simulink model "rev0BB"  (R2017b)
settings: Solver=FixedStepDiscrete  StartTime=0  StopTime=(((preLen+100+dataLenSymbols)*1+pad_first*3)*basePer)  RelTol=1e-3
values from neighbouring files (symbols this model uses):
  ack_stf_len_symbols = length(x_ACK_STF)    [rev0BB_setup.m]
  agc_delay_lag = 32    [rev0BB_setup.m]
  agc_detector_coef = ones(1,agc_detector_taps)./agc_detector_taps    [rev0BB_setup.m]
  agc_on = true    [rev0BB_startup.m]
  agc_sat_low = -agcSaturation    (= -12)    [rev0BB_setup.m]
  agc_sat_up = agcSaturation    (= 12)    [rev0BB_setup.m]
  agcDesired = 0    [rev0BB_setup.m]
  agcExpDomain = agcSaturation    (= 12)    [rev0BB_setup.m]
  agcExpResolution = 2^-5    (= 0.03125)    [rev0BB_setup.m]
  agcPwrAvgNum = 128    [rev0BB_setup.m]
  agcSaturation = 12    [rev0BB_setup.m]
  agcSettleThresh = 0.65    [rev0BB_setup.m]
  agcStep = 2^-8    (= 0.00390625)    [rev0BB_setup.m]
  atanDomain = 5    [rev0BB_setup.m]
  atanDomainTiming = 256    [rev0BB_setup.m]
  atanResolution = 2^-9    (= 0.001953125)    [rev0BB_setup.m]
  atanResolutionTiming = 2^-5    (= 0.03125)    [rev0BB_setup.m]
  averaging_num = ones(1, averaging_samples)    [rev0BB_setup.m]
  averaging_samples = 128    [rev0BB_setup.m]
  awgnSeed = abs(dBSnrRange(dBSnrInd)*1000+trial+10000000)    [plotBer.m]    (also in rev0BB_startup.m = 67)
  basePer = 1/baseFreq    (= 5e-08)    [rev0BB_setup.m]
  bitsPerSymbolHeader = log2(radixHeader)    [rev0BB_setup.m]
  bitsPerSymbolMax = log2(radixMax)    [rev0BB_setup.m]
  cal_sig_i_mult = 1.0    (= 1)    [rev0BB_startup.m]
  cal_sig_i_offset = 0.0    (= 0)    [rev0BB_startup.m]
  cal_sig_q_mult = 1.0    (= 1)    [rev0BB_startup.m]
  cal_sig_q_offset = 0.0    (= 0)    [rev0BB_startup.m]
  cefEarlyWarning = 256    [rev0BB_setup.m]
  cefLen = length(x_CEF)    [rev0BB_setup.m]
  channelFIR = zeros(1, round(maxSampleDelay)+1)    [rev0BB_startup.m]
  coarseCFOAdaptDelay = 1    [rev0BB_setup.m]
  cr_i = 0.020    (= 0.02)    [rev0BB_setup.m]
  cr_i_preamp = 2^-9    (= 0.001953125)    [rev0BB_setup.m]
  cr_int1_sat_low = -cr_integrator1_saturation    (= -0.6)    [rev0BB_setup.m]
  cr_int1_sat_up = cr_integrator1_saturation    (= 0.6)    [rev0BB_setup.m]
  cr_integrator1_decay = 1    [rev0BB_setup.m]
  cr_integrator1_saturation = 0.6    [rev0BB_setup.m]
  cr_mult_pipeline = 0    [rev0BB_setup.m]
  cr_p = 0.015    [rev0BB_setup.m]
  cr_sat2_low = -cr_saturation2    (= -0.6)    [rev0BB_setup.m]
  cr_sat2_up = cr_saturation2    (= 0.6)    [rev0BB_setup.m]
  cr_smooth_num = (1/cr_smooth_samples).*ones(1, cr_smooth_samples)    [rev0BB_setup.m]
  D_128 = [ 1,  8,  2,  4, 16, 32, 64]    [golay.m]    (also in rev0BB_setup.m)
  D_32 = [ 1,  4,  8,  2, 16]    [golay.m]    (also in rev0BB_setup.m)
  dataLenSymbols = header_len_bytes*8/bitsPerSymbolHeader + frame_len_bytes*8/bitsPerSymbol    [rev0BB_setup.m]
  default_channel = 3    [rev0BB_setup.m]
  dmm_coefs = ones(1,dmm_samples)./dmm_samples    [rev0BB_setup.m]
  dst_field_len = 8    [rev0BB_setup.m]
  expDomain = 3.3    [rev0BB_setup.m]
  expResolution = 2^-5    (= 0.03125)    [rev0BB_setup.m]
  expTol = .1    (= 0.1)    [rev0BB_setup.m]
  flush_delay = regular_pipeline*2+mult_pipeline+4    (= 4)    [rev0BB_setup.m]
  frac_lut_domain = 256    [rev0BB_setup.m]
  frac_lut_domain_cr = 64    [rev0BB_setup.m]
  frac_lut_range_max = 512    [rev0BB_setup.m]
  frac_lut_range_max_coarse_cfo = 127    [rev0BB_setup.m]
  frac_lut_range_max_cr = 127    [rev0BB_setup.m]
  frac_lut_range_min = -frac_lut_range_max    (= -512)    [rev0BB_setup.m]
  frac_lut_range_min_coarse_cfo = -frac_lut_range_max_coarse_cfo    (= -127)    [rev0BB_setup.m]
  frac_lut_range_min_cr = -frac_lut_range_max_cr    (= -127)    [rev0BB_setup.m]
  frac_lut_table_breaks = -frac_lut_domain:frac_lut_res:(frac_lut_domain-1)    [rev0BB_setup.m]
  frac_lut_table_breaks_coarse_cfo = -frac_lut_domain_coarse_cfo:frac_lut_res_coarse_cfo:(frac_lut_domain_coarse_cfo-1)    [rev0BB_setup.m]
  frac_lut_table_breaks_cr = -frac_lut_domain_cr:frac_lut_res_cr:(frac_lut_domain_cr-1)    [rev0BB_setup.m]
  frac_lut_table_data = 1./frac_lut_table_breaks    [rev0BB_setup.m]
  frac_lut_table_data_coarse_cfo = 1./frac_lut_table_breaks_coarse_cfo    [rev0BB_setup.m]
  frac_lut_table_data_cr = 1./frac_lut_table_breaks_cr    [rev0BB_setup.m]
  freeze_en_agc = true    [rev0BB_startup.m]
  freeze_en_cr_int1 = false    [rev0BB_startup.m]
  freeze_en_cr_int2 = false    [rev0BB_startup.m]
  freeze_en_cr_phase = false    [rev0BB_startup.m]
  freeze_en_tr_int1 = false    [rev0BB_startup.m]
  freeze_en_tr_int2 = false    [rev0BB_startup.m]
  freeze_en_tr_phase = false    [rev0BB_startup.m]
  freeze_on_cef_done = true    [rev0BB_startup.m]
  freeze_on_stf_done = false    [rev0BB_startup.m]
  freeze_on_valid = true    [rev0BB_startup.m]
  golay_type = 32    [rev0BB_setup.m]
  guardInt = int16(4)    [rev0BB_setup.m]
  guardTol = int16(5)    [rev0BB_setup.m]
  header_len_bytes = 8    [rev0BB_setup.m]
  lineWidth = 60    [rev0BB_setup.m]
  lmsEqDepth = 38    [rev0BB_setup.m]
  lmsStep_init = 0.006    [rev0BB_setup.m]
  lmsStep_meta = (lmsStep_final - lmsStep_init)/cefLen    [rev0BB_setup.m]
  lnDomain = 16    [rev0BB_setup.m]
  lnResolution = 2^-5    (= 0.03125)    [rev0BB_setup.m]
  local_node_id = 2    [rev0BB_startup.m]
  maxMsgSize = length(xSpectrum_PRE)+dataLenSymbols+300    [rev0BB_setup.m]
  minSTFPeaks = 3    [rev0BB_setup.m]
  mod_scheme_len_bytes = 1    [rev0BB_setup.m]
  modBPS = [1, 2, 4]    [rev0BB_setup.m]
  modKeys = [0, 1, 2]    [rev0BB_setup.m]
  mult_pipeline = 0    [rev0BB_setup.m]
  overSampleFreq = 80e6    (= 80000000)    [rev0BB_setup.m]
  overSamplePer = 1/overSampleFreq    (= 1.25e-08)    [rev0BB_setup.m]
  pad_first = 1000    [createTestVectors.m]
  post_cr_i_offset = 0    [rev0BB_startup.m]
  post_cr_q_offset = 0    [rev0BB_startup.m]
  preambleSequentialDetect = 2    [rev0BB_setup.m]
  preLen = length(x_PRE)    [rev0BB_setup.m]
  qam16_demod_scale_factor = qam16_hdl_distance/qam16_power_normalized_distance    [rev0BB_setup.m]
  rcRxFilt = [0.000303163120401141 -0.00118915940834234 -0.00187387637177 -0.00124167532697737 0.00029186889076529 0.00164526160586517 0.00182432050803312 0.000652133621739543 -0.00105668254004908 -0.00204011570659167 -0.00150058088768918 0.00026138356356816 0.0019831869994874 0.00231075800085521 0.000821993419120097 -0.00154687337975486 -0.00305430783933469 -0.00238186490079127 0.000301216962040692 0.00325307 ...(+2001 chars)    [rev0BB_setup.m]
  rcTxFilt = [0.000303163120401141 -0.00118915940834234 -0.00187387637177 -0.00124167532697737 0.00029186889076529 0.00164526160586517 0.00182432050803312 0.000652133621739543 -0.00105668254004908 -0.00204011570659167 -0.00150058088768918 0.00026138356356816 0.0019831869994874 0.00231075800085521 0.000821993419120097 -0.00154687337975486 -0.00305430783933469 -0.00238186490079127 0.000301216962040692 0.00325307 ...(+2001 chars)    [rev0BB_setup.m]
  regular_pipeline = 0    [rev0BB_setup.m]
  rx_gain = 1    [rev0BB_setup.m]
  rx_gain_i = 1    [rev0BB_setup.m]
  rx_gain_q = 1    [rev0BB_setup.m]
  rx_impare_i_offset = 0    [rev0BB_startup.m]
  rx_impare_i_scale = 1    [rev0BB_startup.m]
  rx_impare_q_offset = 0    [rev0BB_startup.m]
  rx_impare_q_scale = 1    [rev0BB_startup.m]
  rx_offset_correction_i = 0    [rev0BB_startup.m]
  rx_offset_correction_q = 0    [rev0BB_startup.m]
  sin_source_amp = 1    [rev0BB_setup.m]
  sin_source_freq = 250e6/16    (= 15625000)    [rev0BB_setup.m]
  slowPer = overSamplePer*slowSample    (= 2.5e-08)    [rev0BB_setup.m]
  std_pkt_type = 0    [rev0BB_setup.m]
  stfLen = length(x_STF)    [rev0BB_setup.m]
  testMsg = cat(1, xCTRL_PRE_adj, header, payload)    [plotBer.m]
  timing_i = 0.25    [rev0BB_setup.m]
  ... (+25 more)
undefined symbols (not defined in the file or in its folder): cr_integrator2_saturation, doppler, i, magnitude, useFadingChannel
libraries: helperLib x128, simulink x90, golayLib x34, dspsigops x32, commfilt2 x27, commdigbbndpm3 x8, hdlsllib x6, dsparch4 x4, commdigbbndam3 x4, commchan3 x2, commrflib2 x2, commcrc2 x2
(part 5 of 10)

== system rev0BB/receiver/fast_rx_baseband/Timing Recovery/SampleAccum ==
  note: Based on Digital Communication Recievers by Meyr pg 530 but modified
      |
      | The error here is in "samples". The correction input is in fact -error and
      | dictates how the clock should be changed.
      |
      | The clk_per is not simply the integer portion of the delay, which is
      | somewhat counterintuitive. This is because the clk_per line is controling
      | the delay for the rx clk (in terms of samples). Here is some intuition:
      | Say that the desired phase is exactly on a sample (fractional delay = 0).
      | One can get the same phase by setting the fractional phase to 1 but the
      | clock must add 1 sample to catch up with the additional delay added.
      |
      | The same logic holds true in the reverse case. Delay can be changed
      | from 1 to 0 but the clock must skip a sample to catch up.
      |
      | Diagrams showing the clock logic as well as the logic when a phase correction
      | is non-zeros are presented to the left of this text.
  note: Division Represented as Shift
  correction : Inport
  Enable : EnablePort
  Add1 : Sum  OutDataTypeStr=Inherit: Same as first input
  Add2 : Sum  OutDataTypeStr=Inherit: Same as first input
  Add4 : Sum  OutDataTypeStr=Inherit: Same as first input
  Constant3 : Constant  Value=4  OutDataTypeStr=Inherit: Inherit via back propagation  SampleTime=-1
  Constant4 : Constant  Value=4  OutDataTypeStr=Inherit: Inherit via back propagation  SampleTime=-1
  Data Type Conversion1 : DataTypeConversion  OutDataTypeStr=int8
  Data Type Conversion2 : DataTypeConversion
  Data Type Conversion3 : DataTypeConversion
  Delay2 : Delay  DelayLength=1  InitialCondition=0
  Gain : Gain  Gain=-1  OutDataTypeStr=Inherit: Same as input
  Sub2 : Sum  Inputs=+-  OutDataTypeStr=Inherit: Same as first input
  Sub3 : Sum  Inputs=+-  OutDataTypeStr=Inherit: Same as first input
  fracDelay : Outport  InitialOutput=[0]
  clk_per : Outport  Port=2  InitialOutput=[0]
  fullDelay : Outport  Port=3  InitialOutput=[0]
  wires:
  Sub3/1 -> Gain/1
  Constant3/1 -> Add1/2
  Data Type Conversion1/1 -> Sub3/1, Data Type Conversion2/1
  Delay2/1 -> Add2/2
  Add2/1 -> fullDelay/1, Data Type Conversion3/1, Data Type Conversion1/1
  Add4/1 -> clk_per/1
  Constant4/1 -> Add4/2, Sub3/2
  correction/1 -> Add1/1
  Gain/1 -> Add4/1
  Sub2/1 -> fracDelay/1, Delay2/1
  Add1/1 -> Add2/1
  Data Type Conversion2/1 -> Sub2/2
  Data Type Conversion3/1 -> Sub2/1

== system rev0BB/receiver/fast_rx_baseband/Timing Recovery/frac_delay_farrow_N-2_M-3 ==
  note: 1
  note: 3
  note: 1
  note: 3
  note: 1
  note: 3
  note: Based on Digital Communication Receivers by Meyr pg 515, 521-522
  note: Delays contained in FIR
  samples : Inport
  delay : Inport  Port=2
  Add : Sum  OutDataTypeStr=Inherit: Same as first input
  Add1 : Sum  OutDataTypeStr=Inherit: Same as first input
  Add2 : Sum  OutDataTypeStr=Inherit: Same as first input
  Discrete FIR Filter : DiscreteFir  FilterStructure=Direct form transposed  Coefficients=[-0.22485, 0.64567, -0.64567, 0.22485]  OutDataTypeStr=Inherit: Same as input
  Discrete FIR Filter1 : DiscreteFir  FilterStructure=Direct form transposed  Coefficients=[0.70609, -1.31155, 0.62547, 0.03154]  OutDataTypeStr=Inherit: Same as input
  Discrete FIR Filter2 : DiscreteFir  FilterStructure=Direct form transposed  Coefficients=[-0.48124, -0.33413, 1.02020, -0.25639]  OutDataTypeStr=Inherit: Same as input
  Discrete FIR Filter3 : DiscreteFir  FilterStructure=Direct form transposed  Coefficients=[0, 1, 0, 0]  OutDataTypeStr=Inherit: Same as input
  Product1 : Product  OutDataTypeStr=Inherit: Same as first input
  Product2 : Product  OutDataTypeStr=Inherit: Same as first input
  Product5 : Product  OutDataTypeStr=Inherit: Same as first input
  mult_delay{,1..5} (6 alike) : Delay  DelayLength=mult_pipeline
  mult_delay_match : Delay  DelayLength=mult_pipeline
  mult_delay_match1 : Delay  DelayLength=mult_pipeline
  mult_delay_match2 : Delay  DelayLength=mult_pipeline
  mult_delay_match3 : Delay  DelayLength=mult_pipeline*2
  mult_delay_match4 : Delay  DelayLength=mult_pipeline*3
  pipeline_delay{,1..10} (11 alike) : Delay  DelayLength=regular_pipeline
  pipeline_delay_match : Delay  DelayLength=regular_pipeline
  pipeline_delay_match1 : Delay  DelayLength=regular_pipeline
  pipeline_delay_match2 : Delay  DelayLength=regular_pipeline
  pipeline_delay_match3 : Delay  DelayLength=regular_pipeline*2
  out : Outport
  wires:
  Discrete FIR Filter3/1 -> pipeline_delay9/1
  Discrete FIR Filter/1 -> pipeline_delay6/1
  delay/1 -> mult_delay3/1, mult_delay_match/1
  samples/1 -> pipeline_delay10/1
  Discrete FIR Filter1/1 -> pipeline_delay7/1
  Product5/1 -> pipeline_delay3/1
  Add/1 -> mult_delay1/1
  Discrete FIR Filter2/1 -> pipeline_delay8/1
  Add1/1 -> mult_delay2/1
  Add2/1 -> out/1
  Product1/1 -> pipeline_delay4/1
  Product2/1 -> pipeline_delay5/1
  mult_delay_match/1 -> pipeline_delay_match/1
  mult_delay_match1/1 -> pipeline_delay_match1/1
  mult_delay_match2/1 -> pipeline_delay/1
  mult_delay_match3/1 -> pipeline_delay_match2/1
  mult_delay_match4/1 -> pipeline_delay_match3/1
  mult_delay3/1 -> Product5/2
  mult_delay/1 -> Product5/1
  mult_delay1/1 -> Product1/1
  mult_delay4/1 -> Product1/2
  mult_delay2/1 -> Product2/1
  mult_delay5/1 -> Product2/2
  pipeline_delay/1 -> Add/1
  pipeline_delay3/1 -> Add/2
  pipeline_delay4/1 -> Add1/2
  pipeline_delay5/1 -> Add2/2
  pipeline_delay_match/1 -> mult_delay_match1/1, mult_delay4/1
  pipeline_delay_match1/1 -> mult_delay5/1
  pipeline_delay6/1 -> mult_delay/1
  pipeline_delay7/1 -> mult_delay_match2/1
  pipeline_delay8/1 -> mult_delay_match3/1
  pipeline_delay9/1 -> mult_delay_match4/1
  pipeline_delay10/1 -> Discrete FIR Filter/1, Discrete FIR Filter1/1, Discrete FIR Filter2/1, Discrete FIR Filter3/1
  pipeline_delay1/1 -> Add1/1
  pipeline_delay_match2/1 -> pipeline_delay1/1
  pipeline_delay2/1 -> Add2/1
  pipeline_delay_match3/1 -> pipeline_delay2/1

== system rev0BB/receiver/fast_rx_baseband/Timing Recovery/loopFilter ==
  In : Inport
  timing_p : Inport  Port=2
  timing_i : Inport  Port=3
  timing_integrator1_decay : Inport  Port=4
  tr_int1_sat_up : Inport  Port=5
  tr_int1_sat_low : Inport  Port=6
  int1_freeze : Inport  Port=7  OutDataTypeStr=boolean
  timing_pre_scale : Inport  Port=8
  tr_sat2_up : Inport  Port=9
  tr_sat2_low : Inport  Port=10
  Enable : EnablePort
  Add : Sum  OutDataTypeStr=Inherit: Same as first input
  Add1 : Sum  OutDataTypeStr=Inherit: Same as first input
  Constant : Constant  Value=0  OutDataTypeStr=Inherit: Inherit via back propagation  SampleTime=-1
  Data Type Duplicate{,1..2,4} (4 alike) : DataTypeDuplicate
  Data Type Conversion4 : DataTypeConversion  OutDataTypeStr=single
  Delay1 : Delay  DelayLength=1  InitialCondition=0
  Delay12 : Delay  DelayLength=1
  Discrete FIR Filter : DiscreteFir  FilterStructure=Direct form transposed  Coefficients=timing_smooth_num  OutDataTypeStr=Inherit: Same as input
  Switch1 : Switch  Criteria=u2 > Threshold
  Switch2 : Switch  Criteria=u2 > Threshold
  pipeline_delay1 : Delay  DelayLength=regular_pipeline
  pipeline_delay5 : Delay  DelayLength=regular_pipeline
  pipeline_delay9 : Delay  DelayLength=regular_pipeline
  pipelined_mult{,1..3} (4 alike) : helperLib/pipelined_mult  d=wide_mult_pipeline
  sat : Subsystem
  sat1 : Subsystem
  Out : Outport  InitialOutput=0
  wires:
  In/1 -> pipeline_delay5/1
  Discrete FIR Filter/1 -> pipeline_delay1/1
  Add/1 -> sat/1(In1)
  sat1/1(Out1) -> Data Type Conversion4/1
  pipelined_mult3/1 -> Switch1/3
  Data Type Conversion4/1 -> Out/1
  pipelined_mult2/1 -> Delay12/1
  Switch2/1 -> Add1/1
  timing_p/1 -> Data Type Duplicate4/1, Data Type Duplicate4/2, pipelined_mult1/2
  timing_integrator1_decay/1 -> Data Type Duplicate/2, pipelined_mult2/1
  timing_i/1 -> pipelined_mult3/2, Data Type Duplicate1/2
  Add1/1 -> pipeline_delay9/1
  tr_int1_sat_up/1 -> sat/2(limit_up)
  tr_int1_sat_low/1 -> sat/3(limit_low)
  Delay1/1 -> Switch1/1
  int1_freeze/1 -> Switch2/2, Switch1/2
  Switch1/1 -> Delay1/1, Add1/2
  pipelined_mult1/1 -> Switch2/3
  Constant/1 -> Switch2/1
  sat/1(Out1) -> Data Type Duplicate1/1, pipelined_mult3/1, Data Type Duplicate/1, pipelined_mult2/2
  pipeline_delay1/1 -> pipelined_mult/1, Data Type Duplicate2/1, pipelined_mult1/1
  timing_pre_scale/1 -> Data Type Duplicate2/2, pipelined_mult/2
  pipeline_delay5/1 -> Discrete FIR Filter/1
  pipelined_mult/1 -> Add/1
  tr_sat2_up/1 -> sat1/2(limit_up)
  tr_sat2_low/1 -> sat1/3(limit_low)
  pipeline_delay9/1 -> sat1/1(In1)
  Delay12/1 -> Add/2

== system rev0BB/receiver/fast_rx_baseband/Timing Recovery/nda_4x_time_err_enable ==
  note: Design from Digital Communication Recievers by Meyr. pg 291, 529
  samples : Inport
  enable : Inport  Port=2
  phase_est : Subsystem
  "tapped_delay4 " : Subsystem  AncestorBlock=helperLib/tapped_delay4
  err : Outport
  wires:
  "tapped_delay4 "/3(delay_1) -> phase_est/3(In3)
  "tapped_delay4 "/4(delay_0) -> phase_est/4(In4)
  "tapped_delay4 "/1(delay_3) -> phase_est/1(In1)
  "tapped_delay4 "/2(delay_2) -> phase_est/2(In2)
  phase_est/1(Out1) -> err/1
  enable/1 -> phase_est/Enable
  samples/1 -> "tapped_delay4 "/1(symbol)

== system rev0BB/receiver/fast_rx_baseband/Timing Recovery/sat ==
  In1 : Inport
  Saturation : Saturate  UpperLimit=.5  LowerLimit=-.5
  Out1 : Outport
  wires:
  Saturation/1 -> Out1/1
  In1/1 -> Saturation/1

== system rev0BB/receiver/slim_fast_rx/AGC/exp ==
  note: Bound Protection
  In : Inport
  Compare To Constant1 : simulink/Logic and Bit Operations/Compare To Constant  relop=>=  const=agcExpDomain  OutDataTypeStr=boolean
  Compare To Constant4 : simulink/Logic and Bit Operations/Compare To Constant  relop=<=  const=-agcExpDomain  OutDataTypeStr=boolean
  Constant11 : Constant  Value=0  OutDataTypeStr=Inherit: Inherit via back propagation  SampleTime=-1
  Constant3 : Constant  Value=exp(agcExpDomain)  OutDataTypeStr=Inherit: Inherit via back propagation  SampleTime=-1
  Constant4 : Constant  Value=exp(-agcExpDomain)  OutDataTypeStr=Inherit: Inherit via back propagation  SampleTime=-1
  Data Type Duplicate : DataTypeDuplicate
  Data Type Duplicate1 : DataTypeDuplicate
  Data Type Duplicate2 : DataTypeDuplicate
  Data Type Conversion : DataTypeConversion  OutDataTypeStr=fixdt(1,ceil(log2(agcExpDomain))-floor(log2(agcExpResolution))+2,-floor(log2(agcExpResolution)))
  Logical Operator : Logic  Operator=OR  AllPortsSameDT=off  OutDataTypeStr=boolean
  Switch2 : Switch  Criteria=u2 ~= 0  OutDataTypeStr=Inherit: Inherit via back propagation
  Switch3 : Switch  Criteria=u2 ~= 0  OutDataTypeStr=Inherit: Inherit via back propagation
  Switch8 : Switch  Criteria=u2 ~= 0  OutDataTypeStr=Inherit: Inherit via back propagation
  exp Lookup Table : Lookup_n-D  NumberOfTableDimensions=1  BreakpointsForDimension1=[-agcExpDomain:agcExpResolution:agcExpDomain]  IndexSearchMethod=Evenly spaced points  Table=exp([-agcExpDomain:agcExpResolution:agcExpDomain])  InterpMethod=Flat  DiagnosticForOutOfRangeInput=Error  RemoveProtectionInput=on  InternalRulePriority=Speed  OutDataTypeStr=Inherit: Inherit via back propagation  RndMeth=Simplest  InputSameDT=on
  pipeline_delay1 : Delay  DelayLength=regular_pipeline
  pipeline_delay2 : Delay  DelayLength=regular_pipeline  InitialCondition=1
  pipeline_delay_match : Delay  DelayLength=regular_pipeline*2
  pipeline_delay_match1 : Delay  DelayLength=regular_pipeline*2
  Out : Outport
  wires:
  pipeline_delay2/1 -> Data Type Duplicate2/1, Switch2/3
  pipeline_delay1/1 -> exp Lookup Table/1
  pipeline_delay_match1/1 -> Switch3/2
  pipeline_delay_match/1 -> Switch2/2
  exp Lookup Table/1 -> Data Type Duplicate/2, pipeline_delay2/1
  Constant11/1 -> Switch8/1
  Logical Operator/1 -> Switch8/2
  Switch3/1 -> Data Type Duplicate1/2, Data Type Duplicate2/2, Out/1
  Constant4/1 -> Switch3/1
  Switch2/1 -> Data Type Duplicate1/1, Switch3/3
  Constant3/1 -> Switch2/1
  Compare To Constant4/1 -> pipeline_delay_match1/1, Logical Operator/2
  Compare To Constant1/1 -> pipeline_delay_match/1, Logical Operator/1
  In/1 -> Data Type Duplicate/1, Compare To Constant4/1, Compare To Constant1/1, Switch8/3
  Switch8/1 -> Data Type Conversion/1
  Data Type Conversion/1 -> pipeline_delay1/1

== system rev0BB/receiver/slim_fast_rx/AGC/exp1 ==
  note: Bound Protection
  In : Inport
  Compare To Constant1 : simulink/Logic and Bit Operations/Compare To Constant  relop=>=  const=agcExpDomain*2  OutDataTypeStr=boolean
  Compare To Constant4 : simulink/Logic and Bit Operations/Compare To Constant  relop=<=  const=-agcExpDomain*2  OutDataTypeStr=boolean
  Constant11 : Constant  Value=0  OutDataTypeStr=Inherit: Inherit via back propagation  SampleTime=-1
  Constant3 : Constant  Value=exp(agcExpDomain*2)  OutDataTypeStr=Inherit: Inherit via back propagation  SampleTime=-1
  Constant4 : Constant  Value=exp(-agcExpDomain)  OutDataTypeStr=Inherit: Inherit via back propagation  SampleTime=-1
  Data Type Duplicate : DataTypeDuplicate
  Data Type Duplicate1 : DataTypeDuplicate
  Data Type Duplicate2 : DataTypeDuplicate
  Data Type Conversion : DataTypeConversion  OutDataTypeStr=fixdt(1,ceil(log2(agcExpDomain*2))-floor(log2(agcExpResolution))+2,-floor(log2(agcExpResolution)))
  Logical Operator : Logic  Operator=OR  AllPortsSameDT=off  OutDataTypeStr=boolean
  Switch2 : Switch  Criteria=u2 ~= 0  OutDataTypeStr=Inherit: Inherit via back propagation
  Switch3 : Switch  Criteria=u2 ~= 0  OutDataTypeStr=Inherit: Inherit via back propagation
  Switch8 : Switch  Criteria=u2 ~= 0  OutDataTypeStr=Inherit: Inherit via back propagation
  exp Lookup Table : Lookup_n-D  NumberOfTableDimensions=1  BreakpointsForDimension1=[(-agcExpDomain*2):agcExpResolution:agcExpDomain*2]  IndexSearchMethod=Evenly spaced points  Table=exp([(-agcExpDomain*2):agcExpResolution:(agcExpDomain*2)])  InterpMethod=Flat  DiagnosticForOutOfRangeInput=Error  RemoveProtectionInput=on  InternalRulePriority=Speed  OutDataTypeStr=Inherit: Inherit via back propagation  RndMeth=Simplest  InputSameDT=on
  mult_delay : Delay  DelayLength=wide_mult_pipeline
  mult_delay_match : Delay  DelayLength=wide_mult_pipeline
  mult_delay_match1 : Delay  DelayLength=wide_mult_pipeline
  pipeline_delay1 : Delay  DelayLength=regular_pipeline
  pipeline_delay2 : Delay  DelayLength=regular_pipeline  InitialCondition=1
  pipeline_delay_match : Delay  DelayLength=regular_pipeline*2
  pipeline_delay_match1 : Delay  DelayLength=regular_pipeline*2
  Out : Outport
  wires:
  pipeline_delay2/1 -> Switch2/3, Data Type Duplicate2/2
  mult_delay/1 -> exp Lookup Table/1
  pipeline_delay1/1 -> mult_delay/1
  mult_delay_match1/1 -> Switch3/2
  mult_delay_match/1 -> Switch2/2
  pipeline_delay_match1/1 -> mult_delay_match1/1
  pipeline_delay_match/1 -> mult_delay_match/1
  exp Lookup Table/1 -> Data Type Duplicate/2, pipeline_delay2/1
  Switch8/1 -> Data Type Conversion/1
  Constant11/1 -> Switch8/1
  Logical Operator/1 -> Switch8/2
  Switch3/1 -> Data Type Duplicate2/1, Data Type Duplicate1/2, Out/1
  Constant4/1 -> Switch3/1
  Switch2/1 -> Data Type Duplicate1/1, Switch3/3
  Constant3/1 -> Switch2/1
  Compare To Constant4/1 -> pipeline_delay_match1/1, Logical Operator/2
  Compare To Constant1/1 -> pipeline_delay_match/1, Logical Operator/1
  In/1 -> Data Type Duplicate/1, Compare To Constant4/1, Compare To Constant1/1, Switch8/3
  Data Type Conversion/1 -> pipeline_delay1/1

== system rev0BB/receiver/slim_fast_rx/AGC/ln1 ==
  note: Note that output type is scaled back
  note: Bound Protection
  In : Inport
  data_type : Inport  Port=2
  Compare To Constant1 : simulink/Logic and Bit Operations/Compare To Constant  relop=>=  const=lnDomain  OutDataTypeStr=boolean
  Compare To Constant4 : simulink/Logic and Bit Operations/Compare To Constant  relop=<=  const=lnResolution  OutDataTypeStr=boolean
  Constant11 : Constant  Value=lnResolution  OutDataTypeStr=Inherit: Inherit via back propagation  SampleTime=-1
  Constant3 : Constant  Value=log(lnDomain)  OutDataTypeStr=Inherit: Inherit via back propagation  SampleTime=-1
  Constant4 : Constant  Value=log(lnResolution)  OutDataTypeStr=Inherit: Inherit via back propagation  SampleTime=-1
  Data Type Duplicate : DataTypeDuplicate
  Data Type Conversion : DataTypeConversion  OutDataTypeStr=single
  Logical Operator : Logic  Operator=OR  AllPortsSameDT=off  OutDataTypeStr=boolean
  Saturation : Saturate  UpperLimit=lnDomain  LowerLimit=lnResolution
  Switch2 : Switch  Criteria=u2 ~= 0  OutDataTypeStr=Inherit: Inherit via back propagation
  Switch3 : Switch  Criteria=u2 ~= 0  OutDataTypeStr=Inherit: Inherit via back propagation
  Switch8 : Switch  Criteria=u2 ~= 0  OutDataTypeStr=Inherit: Inherit via back propagation
  ln Lookup Table : Lookup_n-D  NumberOfTableDimensions=1  BreakpointsForDimension1=[lnResolution:lnResolution:lnDomain]  IndexSearchMethod=Evenly spaced points  Table=log([lnResolution:lnResolution:lnDomain])  InterpMethod=Flat  DiagnosticForOutOfRangeInput=Error  RemoveProtectionInput=on  InternalRulePriority=Speed  OutDataTypeStr=Inherit: Inherit via back propagation  RndMeth=Simplest  InputSameDT=on
  pipeline_delay1 : Delay  DelayLength=regular_pipeline  InitialCondition=0
  pipeline_delay2 : Delay  DelayLength=regular_pipeline*2
  pipeline_delay3 : Delay  DelayLength=regular_pipeline*1  InitialCondition=1
  pipeline_delay_match : Delay  DelayLength=regular_pipeline*4
  pipeline_delay_match1 : Delay  DelayLength=regular_pipeline*4
  Out : Outport
  wires:
  pipeline_delay2/1 -> Switch2/3
  pipeline_delay1/1 -> Saturation/1
  pipeline_delay_match1/1 -> Switch3/2
  pipeline_delay_match/1 -> Switch2/2
  ln Lookup Table/1 -> Data Type Duplicate/2, pipeline_delay2/1
  Constant11/1 -> Switch8/1
  Logical Operator/1 -> Switch8/2
  Switch3/1 -> Out/1
  Constant4/1 -> Switch3/1
  Switch2/1 -> Switch3/3
  Constant3/1 -> Switch2/1
  Compare To Constant4/1 -> pipeline_delay_match1/1, Logical Operator/2
  Compare To Constant1/1 -> pipeline_delay_match/1, Logical Operator/1
  Saturation/1 -> pipeline_delay3/1
  pipeline_delay3/1 -> ln Lookup Table/1
  In/1 -> Compare To Constant4/1, Compare To Constant1/1, Switch8/3
  data_type/1 -> Data Type Duplicate/1
  Switch8/1 -> Data Type Conversion/1
  Data Type Conversion/1 -> pipeline_delay1/1

== system rev0BB/receiver/slim_fast_rx1/AGC/exp ==
  note: Bound Protection
  In : Inport
  Compare To Constant1 : simulink/Logic and Bit Operations/Compare To Constant  relop=>=  const=agcExpDomain  OutDataTypeStr=boolean
  Compare To Constant4 : simulink/Logic and Bit Operations/Compare To Constant  relop=<=  const=-agcExpDomain  OutDataTypeStr=boolean
  Constant11 : Constant  Value=0  OutDataTypeStr=Inherit: Inherit via back propagation  SampleTime=-1
  Constant3 : Constant  Value=exp(agcExpDomain)  OutDataTypeStr=Inherit: Inherit via back propagation  SampleTime=-1
  Constant4 : Constant  Value=exp(-agcExpDomain)  OutDataTypeStr=Inherit: Inherit via back propagation  SampleTime=-1
  Data Type Duplicate : DataTypeDuplicate
  Data Type Duplicate1 : DataTypeDuplicate
  Data Type Duplicate2 : DataTypeDuplicate
  Data Type Conversion : DataTypeConversion  OutDataTypeStr=fixdt(1,ceil(log2(agcExpDomain))-floor(log2(agcExpResolution))+2,-floor(log2(agcExpResolution)))
  Logical Operator : Logic  Operator=OR  AllPortsSameDT=off  OutDataTypeStr=boolean
  Switch2 : Switch  Criteria=u2 ~= 0  OutDataTypeStr=Inherit: Inherit via back propagation
  Switch3 : Switch  Criteria=u2 ~= 0  OutDataTypeStr=Inherit: Inherit via back propagation
  Switch8 : Switch  Criteria=u2 ~= 0  OutDataTypeStr=Inherit: Inherit via back propagation
  exp Lookup Table : Lookup_n-D  NumberOfTableDimensions=1  BreakpointsForDimension1=[-agcExpDomain:agcExpResolution:agcExpDomain]  IndexSearchMethod=Evenly spaced points  Table=exp([-agcExpDomain:agcExpResolution:agcExpDomain])  InterpMethod=Flat  DiagnosticForOutOfRangeInput=Error  RemoveProtectionInput=on  InternalRulePriority=Speed  OutDataTypeStr=Inherit: Inherit via back propagation  RndMeth=Simplest  InputSameDT=on
  pipeline_delay1 : Delay  DelayLength=regular_pipeline
  pipeline_delay2 : Delay  DelayLength=regular_pipeline  InitialCondition=1
  pipeline_delay_match : Delay  DelayLength=regular_pipeline*2
  pipeline_delay_match1 : Delay  DelayLength=regular_pipeline*2
  Out : Outport
  wires:
  pipeline_delay2/1 -> Data Type Duplicate2/1, Switch2/3
  pipeline_delay1/1 -> exp Lookup Table/1
  pipeline_delay_match1/1 -> Switch3/2
  pipeline_delay_match/1 -> Switch2/2
  exp Lookup Table/1 -> Data Type Duplicate/2, pipeline_delay2/1
  Constant11/1 -> Switch8/1
  Logical Operator/1 -> Switch8/2
  Switch3/1 -> Data Type Duplicate1/2, Data Type Duplicate2/2, Out/1
  Constant4/1 -> Switch3/1
  Switch2/1 -> Data Type Duplicate1/1, Switch3/3
  Constant3/1 -> Switch2/1
  Compare To Constant4/1 -> pipeline_delay_match1/1, Logical Operator/2
  Compare To Constant1/1 -> pipeline_delay_match/1, Logical Operator/1
  In/1 -> Data Type Duplicate/1, Compare To Constant4/1, Compare To Constant1/1, Switch8/3
  Switch8/1 -> Data Type Conversion/1
  Data Type Conversion/1 -> pipeline_delay1/1

== system rev0BB/receiver/slim_fast_rx1/AGC/exp1 ==
  note: Bound Protection
  In : Inport
  Compare To Constant1 : simulink/Logic and Bit Operations/Compare To Constant  relop=>=  const=agcExpDomain*2  OutDataTypeStr=boolean
  Compare To Constant4 : simulink/Logic and Bit Operations/Compare To Constant  relop=<=  const=-agcExpDomain*2  OutDataTypeStr=boolean
  Constant11 : Constant  Value=0  OutDataTypeStr=Inherit: Inherit via back propagation  SampleTime=-1
  Constant3 : Constant  Value=exp(agcExpDomain*2)  OutDataTypeStr=Inherit: Inherit via back propagation  SampleTime=-1
  Constant4 : Constant  Value=exp(-agcExpDomain)  OutDataTypeStr=Inherit: Inherit via back propagation  SampleTime=-1
  Data Type Duplicate : DataTypeDuplicate
  Data Type Duplicate1 : DataTypeDuplicate
  Data Type Duplicate2 : DataTypeDuplicate
  Data Type Conversion : DataTypeConversion  OutDataTypeStr=fixdt(1,ceil(log2(agcExpDomain*2))-floor(log2(agcExpResolution))+2,-floor(log2(agcExpResolution)))
  Logical Operator : Logic  Operator=OR  AllPortsSameDT=off  OutDataTypeStr=boolean
  Switch2 : Switch  Criteria=u2 ~= 0  OutDataTypeStr=Inherit: Inherit via back propagation
  Switch3 : Switch  Criteria=u2 ~= 0  OutDataTypeStr=Inherit: Inherit via back propagation
  Switch8 : Switch  Criteria=u2 ~= 0  OutDataTypeStr=Inherit: Inherit via back propagation
  exp Lookup Table : Lookup_n-D  NumberOfTableDimensions=1  BreakpointsForDimension1=[(-agcExpDomain*2):agcExpResolution:agcExpDomain*2]  IndexSearchMethod=Evenly spaced points  Table=exp([(-agcExpDomain*2):agcExpResolution:(agcExpDomain*2)])  InterpMethod=Flat  DiagnosticForOutOfRangeInput=Error  RemoveProtectionInput=on  InternalRulePriority=Speed  OutDataTypeStr=Inherit: Inherit via back propagation  RndMeth=Simplest  InputSameDT=on
  mult_delay : Delay  DelayLength=wide_mult_pipeline
  mult_delay_match : Delay  DelayLength=wide_mult_pipeline
  mult_delay_match1 : Delay  DelayLength=wide_mult_pipeline
  pipeline_delay1 : Delay  DelayLength=regular_pipeline
  pipeline_delay2 : Delay  DelayLength=regular_pipeline  InitialCondition=1
  pipeline_delay_match : Delay  DelayLength=regular_pipeline*2
  pipeline_delay_match1 : Delay  DelayLength=regular_pipeline*2
  Out : Outport
  wires:
  pipeline_delay2/1 -> Switch2/3, Data Type Duplicate2/2
  mult_delay/1 -> exp Lookup Table/1
  pipeline_delay1/1 -> mult_delay/1
  mult_delay_match1/1 -> Switch3/2
  mult_delay_match/1 -> Switch2/2
  pipeline_delay_match1/1 -> mult_delay_match1/1
  pipeline_delay_match/1 -> mult_delay_match/1
  exp Lookup Table/1 -> Data Type Duplicate/2, pipeline_delay2/1
  Switch8/1 -> Data Type Conversion/1
  Constant11/1 -> Switch8/1
  Logical Operator/1 -> Switch8/2
  Switch3/1 -> Data Type Duplicate2/1, Data Type Duplicate1/2, Out/1
  Constant4/1 -> Switch3/1
  Switch2/1 -> Data Type Duplicate1/1, Switch3/3
  Constant3/1 -> Switch2/1
  Compare To Constant4/1 -> pipeline_delay_match1/1, Logical Operator/2
  Compare To Constant1/1 -> pipeline_delay_match/1, Logical Operator/1
  In/1 -> Data Type Duplicate/1, Compare To Constant4/1, Compare To Constant1/1, Switch8/3
  Data Type Conversion/1 -> pipeline_delay1/1

== system rev0BB/receiver/slim_fast_rx1/AGC/ln1 ==
  note: Note that output type is scaled back
  note: Bound Protection
  In : Inport
  data_type : Inport  Port=2
  Compare To Constant1 : simulink/Logic and Bit Operations/Compare To Constant  relop=>=  const=lnDomain  OutDataTypeStr=boolean
  Compare To Constant4 : simulink/Logic and Bit Operations/Compare To Constant  relop=<=  const=lnResolution  OutDataTypeStr=boolean
  Constant11 : Constant  Value=lnResolution  OutDataTypeStr=Inherit: Inherit via back propagation  SampleTime=-1
  Constant3 : Constant  Value=log(lnDomain)  OutDataTypeStr=Inherit: Inherit via back propagation  SampleTime=-1
  Constant4 : Constant  Value=log(lnResolution)  OutDataTypeStr=Inherit: Inherit via back propagation  SampleTime=-1
  Data Type Duplicate : DataTypeDuplicate
  Data Type Conversion : DataTypeConversion  OutDataTypeStr=fixdt(1,ceil(log2(lnDomain))-floor(log2(lnResolution))+2,-floor(log2(lnResolution)))
  Logical Operator : Logic  Operator=OR  AllPortsSameDT=off  OutDataTypeStr=boolean
  Saturation : Saturate  UpperLimit=lnDomain  LowerLimit=lnResolution
  Switch2 : Switch  Criteria=u2 ~= 0  OutDataTypeStr=Inherit: Inherit via back propagation
  Switch3 : Switch  Criteria=u2 ~= 0  OutDataTypeStr=Inherit: Inherit via back propagation
  Switch8 : Switch  Criteria=u2 ~= 0  OutDataTypeStr=Inherit: Inherit via back propagation
  ln Lookup Table : Lookup_n-D  NumberOfTableDimensions=1  BreakpointsForDimension1=[lnResolution:lnResolution:lnDomain]  IndexSearchMethod=Evenly spaced points  Table=log([lnResolution:lnResolution:lnDomain])  InterpMethod=Flat  DiagnosticForOutOfRangeInput=Error  RemoveProtectionInput=on  InternalRulePriority=Speed  OutDataTypeStr=Inherit: Inherit via back propagation  RndMeth=Simplest  InputSameDT=on
  pipeline_delay1 : Delay  DelayLength=regular_pipeline  InitialCondition=0
  pipeline_delay2 : Delay  DelayLength=regular_pipeline*2
  pipeline_delay3 : Delay  DelayLength=regular_pipeline*1  InitialCondition=1
  pipeline_delay_match : Delay  DelayLength=regular_pipeline*4
  pipeline_delay_match1 : Delay  DelayLength=regular_pipeline*4
  Out : Outport
  wires:
  pipeline_delay2/1 -> Switch2/3
  pipeline_delay1/1 -> Saturation/1
  pipeline_delay_match1/1 -> Switch3/2
  pipeline_delay_match/1 -> Switch2/2
  ln Lookup Table/1 -> Data Type Duplicate/2, pipeline_delay2/1
  Constant11/1 -> Switch8/1
  Logical Operator/1 -> Switch8/2
  Switch3/1 -> Out/1
  Constant4/1 -> Switch3/1
  Switch2/1 -> Switch3/3
  Constant3/1 -> Switch2/1
  Compare To Constant4/1 -> pipeline_delay_match1/1, Logical Operator/2
  Compare To Constant1/1 -> pipeline_delay_match/1, Logical Operator/1
  Saturation/1 -> pipeline_delay3/1
  pipeline_delay3/1 -> ln Lookup Table/1
  In/1 -> Compare To Constant4/1, Compare To Constant1/1, Switch8/3
  data_type/1 -> Data Type Duplicate/1
  Switch8/1 -> Data Type Conversion/1
  Data Type Conversion/1 -> pipeline_delay1/1

== system rev0BB/receiver/slim_fast_rx1/coarseCFO_direct_ff/RxRaisedCosine ==
  In2 : Inport
  Discrete FIR Filter : DiscreteFir  FilterStructure=Direct form transposed  Coefficients=rcRxFilt  AccumDataTypeStr=Inherit: Same as product output
  Raised Cosine Receive Filter : commfilt2/Raised Cosine Receive Filter  Commented=on  filtType=Square root  R=0.2  filtSpan=40  N=4  downFactor=1  downOffset=0  filterGain=1  InputProcessing=Columns as channels (frame based)  RateOptions=Enforce single-rate processing  framing=Mute  checkCoeff=on  variableName=rcRxFilt  currentFiltSpan=40  D=(40)/2  inputOffset=0  sampMode=Mute  saveAsFlag=0  rateMode=Downsampling  checkGain=Normalized  launchFVT=on  roundingMode=Floor  overflowMode=off  coeffDataTypeStr=Inherit: Same word length as input  coeffMin=[]  coeffMax=[]  coeffLastDataTypeStr=Inherit: Same word length as input  accumDataTypeStr=Inherit: Same as product output  accumLastDataTypeStr=Inherit: Same as product output  outputDataTypeStr=Inherit: Same as accumulator  outputMin=[]  outputMax=[]  outputLastDataTypeStr=Inherit: Same as accumulator
  Out2 : Outport
  wires:
  Discrete FIR Filter/1 -> Out2/1
  In2/1 -> Discrete FIR Filter/1

== system rev0BB/receiver/slim_fast_rx1/coarseCFO_direct_ff/RxRaisedCosine1 ==
  In2 : Inport
  Discrete FIR Filter : DiscreteFir  FilterStructure=Direct form transposed  Coefficients=rcRxFilt  AccumDataTypeStr=Inherit: Same as product output
  Raised Cosine Receive Filter : commfilt2/Raised Cosine Receive Filter  Commented=on  filtType=Square root  R=0.2  filtSpan=40  N=4  downFactor=1  downOffset=0  filterGain=1  InputProcessing=Columns as channels (frame based)  RateOptions=Enforce single-rate processing  framing=Mute  checkCoeff=on  variableName=rcRxFilt  currentFiltSpan=40  D=(40)/2  inputOffset=0  sampMode=Mute  saveAsFlag=0  rateMode=Downsampling  checkGain=Normalized  launchFVT=on  roundingMode=Floor  overflowMode=off  coeffDataTypeStr=Inherit: Same word length as input  coeffMin=[]  coeffMax=[]  coeffLastDataTypeStr=Inherit: Same word length as input  accumDataTypeStr=Inherit: Same as product output  accumLastDataTypeStr=Inherit: Same as product output  outputDataTypeStr=Inherit: Same as accumulator  outputMin=[]  outputMax=[]  outputLastDataTypeStr=Inherit: Same as accumulator
  Out2 : Outport
  wires:
  Discrete FIR Filter/1 -> Out2/1
  In2/1 -> Discrete FIR Filter/1

== system rev0BB/receiver/slim_fast_rx1/coarseCFO_direct_ff/RxRaisedCosine10 ==
  In2 : Inport
  Discrete FIR Filter : DiscreteFir  FilterStructure=Direct form transposed  Coefficients=rcRxFilt  AccumDataTypeStr=Inherit: Same as product output
  Raised Cosine Receive Filter : commfilt2/Raised Cosine Receive Filter  Commented=on  filtType=Square root  R=0.2  filtSpan=40  N=4  downFactor=1  downOffset=0  filterGain=1  InputProcessing=Columns as channels (frame based)  RateOptions=Enforce single-rate processing  framing=Mute  checkCoeff=on  variableName=rcRxFilt  currentFiltSpan=40  D=(40)/2  inputOffset=0  sampMode=Mute  saveAsFlag=0  rateMode=Downsampling  checkGain=Normalized  launchFVT=on  roundingMode=Floor  overflowMode=off  coeffDataTypeStr=Inherit: Same word length as input  coeffMin=[]  coeffMax=[]  coeffLastDataTypeStr=Inherit: Same word length as input  accumDataTypeStr=Inherit: Same as product output  accumLastDataTypeStr=Inherit: Same as product output  outputDataTypeStr=Inherit: Same as accumulator  outputMin=[]  outputMax=[]  outputLastDataTypeStr=Inherit: Same as accumulator
  Out2 : Outport
  wires:
  Discrete FIR Filter/1 -> Out2/1
  In2/1 -> Discrete FIR Filter/1

== system rev0BB/receiver/slim_fast_rx1/coarseCFO_direct_ff/RxRaisedCosine2 ==
  In2 : Inport
  Discrete FIR Filter : DiscreteFir  FilterStructure=Direct form transposed  Coefficients=rcRxFilt  AccumDataTypeStr=Inherit: Same as product output
  Raised Cosine Receive Filter : commfilt2/Raised Cosine Receive Filter  Commented=on  filtType=Square root  R=0.2  filtSpan=40  N=4  downFactor=1  downOffset=0  filterGain=1  InputProcessing=Columns as channels (frame based)  RateOptions=Enforce single-rate processing  framing=Mute  checkCoeff=on  variableName=rcRxFilt  currentFiltSpan=40  D=(40)/2  inputOffset=0  sampMode=Mute  saveAsFlag=0  rateMode=Downsampling  checkGain=Normalized  launchFVT=on  roundingMode=Floor  overflowMode=off  coeffDataTypeStr=Inherit: Same word length as input  coeffMin=[]  coeffMax=[]  coeffLastDataTypeStr=Inherit: Same word length as input  accumDataTypeStr=Inherit: Same as product output  accumLastDataTypeStr=Inherit: Same as product output  outputDataTypeStr=Inherit: Same as accumulator  outputMin=[]  outputMax=[]  outputLastDataTypeStr=Inherit: Same as accumulator
  Out2 : Outport
  wires:
  Discrete FIR Filter/1 -> Out2/1
  In2/1 -> Discrete FIR Filter/1

== system rev0BB/receiver/slim_fast_rx1/coarseCFO_direct_ff/RxRaisedCosine3 ==
  In2 : Inport
  Discrete FIR Filter : DiscreteFir  FilterStructure=Direct form transposed  Coefficients=rcRxFilt  AccumDataTypeStr=Inherit: Same as product output
  Raised Cosine Receive Filter : commfilt2/Raised Cosine Receive Filter  Commented=on  filtType=Square root  R=0.2  filtSpan=40  N=4  downFactor=1  downOffset=0  filterGain=1  InputProcessing=Columns as channels (frame based)  RateOptions=Enforce single-rate processing  framing=Mute  checkCoeff=on  variableName=rcRxFilt  currentFiltSpan=40  D=(40)/2  inputOffset=0  sampMode=Mute  saveAsFlag=0  rateMode=Downsampling  checkGain=Normalized  launchFVT=on  roundingMode=Floor  overflowMode=off  coeffDataTypeStr=Inherit: Same word length as input  coeffMin=[]  coeffMax=[]  coeffLastDataTypeStr=Inherit: Same word length as input  accumDataTypeStr=Inherit: Same as product output  accumLastDataTypeStr=Inherit: Same as product output  outputDataTypeStr=Inherit: Same as accumulator  outputMin=[]  outputMax=[]  outputLastDataTypeStr=Inherit: Same as accumulator
  Out2 : Outport
  wires:
  Discrete FIR Filter/1 -> Out2/1
  In2/1 -> Discrete FIR Filter/1

== system rev0BB/receiver/slim_fast_rx1/coarseCFO_direct_ff/RxRaisedCosine4 ==
  In2 : Inport
  Discrete FIR Filter : DiscreteFir  FilterStructure=Direct form transposed  Coefficients=rcRxFilt  AccumDataTypeStr=Inherit: Same as product output
  Raised Cosine Receive Filter : commfilt2/Raised Cosine Receive Filter  Commented=on  filtType=Square root  R=0.2  filtSpan=40  N=4  downFactor=1  downOffset=0  filterGain=1  InputProcessing=Columns as channels (frame based)  RateOptions=Enforce single-rate processing  framing=Mute  checkCoeff=on  variableName=rcRxFilt  currentFiltSpan=40  D=(40)/2  inputOffset=0  sampMode=Mute  saveAsFlag=0  rateMode=Downsampling  checkGain=Normalized  launchFVT=on  roundingMode=Floor  overflowMode=off  coeffDataTypeStr=Inherit: Same word length as input  coeffMin=[]  coeffMax=[]  coeffLastDataTypeStr=Inherit: Same word length as input  accumDataTypeStr=Inherit: Same as product output  accumLastDataTypeStr=Inherit: Same as product output  outputDataTypeStr=Inherit: Same as accumulator  outputMin=[]  outputMax=[]  outputLastDataTypeStr=Inherit: Same as accumulator
  Out2 : Outport
  wires:
  Discrete FIR Filter/1 -> Out2/1
  In2/1 -> Discrete FIR Filter/1

== system rev0BB/receiver/slim_fast_rx1/coarseCFO_direct_ff/RxRaisedCosine5 ==
  In2 : Inport
  Discrete FIR Filter : DiscreteFir  FilterStructure=Direct form transposed  Coefficients=rcRxFilt  AccumDataTypeStr=Inherit: Same as product output
  Raised Cosine Receive Filter : commfilt2/Raised Cosine Receive Filter  Commented=on  filtType=Square root  R=0.2  filtSpan=40  N=4  downFactor=1  downOffset=0  filterGain=1  InputProcessing=Columns as channels (frame based)  RateOptions=Enforce single-rate processing  framing=Mute  checkCoeff=on  variableName=rcRxFilt  currentFiltSpan=40  D=(40)/2  inputOffset=0  sampMode=Mute  saveAsFlag=0  rateMode=Downsampling  checkGain=Normalized  launchFVT=on  roundingMode=Floor  overflowMode=off  coeffDataTypeStr=Inherit: Same word length as input  coeffMin=[]  coeffMax=[]  coeffLastDataTypeStr=Inherit: Same word length as input  accumDataTypeStr=Inherit: Same as product output  accumLastDataTypeStr=Inherit: Same as product output  outputDataTypeStr=Inherit: Same as accumulator  outputMin=[]  outputMax=[]  outputLastDataTypeStr=Inherit: Same as accumulator
  Out2 : Outport
  wires:
  Discrete FIR Filter/1 -> Out2/1
  In2/1 -> Discrete FIR Filter/1

== system rev0BB/receiver/slim_fast_rx1/coarseCFO_direct_ff/RxRaisedCosine6 ==
  In2 : Inport
  Discrete FIR Filter : DiscreteFir  FilterStructure=Direct form transposed  Coefficients=rcRxFilt  AccumDataTypeStr=Inherit: Same as product output
  Raised Cosine Receive Filter : commfilt2/Raised Cosine Receive Filter  Commented=on  filtType=Square root  R=0.2  filtSpan=40  N=4  downFactor=1  downOffset=0  filterGain=1  InputProcessing=Columns as channels (frame based)  RateOptions=Enforce single-rate processing  framing=Mute  checkCoeff=on  variableName=rcRxFilt  currentFiltSpan=40  D=(40)/2  inputOffset=0  sampMode=Mute  saveAsFlag=0  rateMode=Downsampling  checkGain=Normalized  launchFVT=on  roundingMode=Floor  overflowMode=off  coeffDataTypeStr=Inherit: Same word length as input  coeffMin=[]  coeffMax=[]  coeffLastDataTypeStr=Inherit: Same word length as input  accumDataTypeStr=Inherit: Same as product output  accumLastDataTypeStr=Inherit: Same as product output  outputDataTypeStr=Inherit: Same as accumulator  outputMin=[]  outputMax=[]  outputLastDataTypeStr=Inherit: Same as accumulator
  Out2 : Outport
  wires:
  Discrete FIR Filter/1 -> Out2/1
  In2/1 -> Discrete FIR Filter/1

== system rev0BB/receiver/slim_fast_rx1/coarseCFO_direct_ff/RxRaisedCosine7 ==
  In2 : Inport
  Discrete FIR Filter : DiscreteFir  FilterStructure=Direct form transposed  Coefficients=rcRxFilt  AccumDataTypeStr=Inherit: Same as product output
  Raised Cosine Receive Filter : commfilt2/Raised Cosine Receive Filter  Commented=on  filtType=Square root  R=0.2  filtSpan=40  N=4  downFactor=1  downOffset=0  filterGain=1  InputProcessing=Columns as channels (frame based)  RateOptions=Enforce single-rate processing  framing=Mute  checkCoeff=on  variableName=rcRxFilt  currentFiltSpan=40  D=(40)/2  inputOffset=0  sampMode=Mute  saveAsFlag=0  rateMode=Downsampling  checkGain=Normalized  launchFVT=on  roundingMode=Floor  overflowMode=off  coeffDataTypeStr=Inherit: Same word length as input  coeffMin=[]  coeffMax=[]  coeffLastDataTypeStr=Inherit: Same word length as input  accumDataTypeStr=Inherit: Same as product output  accumLastDataTypeStr=Inherit: Same as product output  outputDataTypeStr=Inherit: Same as accumulator  outputMin=[]  outputMax=[]  outputLastDataTypeStr=Inherit: Same as accumulator
  Out2 : Outport
  wires:
  Discrete FIR Filter/1 -> Out2/1
  In2/1 -> Discrete FIR Filter/1

== system rev0BB/receiver/slim_fast_rx1/coarseCFO_direct_ff/RxRaisedCosine8 ==
  In2 : Inport
  Discrete FIR Filter : DiscreteFir  FilterStructure=Direct form transposed  Coefficients=rcRxFilt  AccumDataTypeStr=Inherit: Same as product output
  Raised Cosine Receive Filter : commfilt2/Raised Cosine Receive Filter  Commented=on  filtType=Square root  R=0.2  filtSpan=40  N=4  downFactor=1  downOffset=0  filterGain=1  InputProcessing=Columns as channels (frame based)  RateOptions=Enforce single-rate processing  framing=Mute  checkCoeff=on  variableName=rcRxFilt  currentFiltSpan=40  D=(40)/2  inputOffset=0  sampMode=Mute  saveAsFlag=0  rateMode=Downsampling  checkGain=Normalized  launchFVT=on  roundingMode=Floor  overflowMode=off  coeffDataTypeStr=Inherit: Same word length as input  coeffMin=[]  coeffMax=[]  coeffLastDataTypeStr=Inherit: Same word length as input  accumDataTypeStr=Inherit: Same as product output  accumLastDataTypeStr=Inherit: Same as product output  outputDataTypeStr=Inherit: Same as accumulator  outputMin=[]  outputMax=[]  outputLastDataTypeStr=Inherit: Same as accumulator
  Out2 : Outport
  wires:
  Discrete FIR Filter/1 -> Out2/1
  In2/1 -> Discrete FIR Filter/1

== system rev0BB/receiver/slim_fast_rx1/coarseCFO_direct_ff/RxRaisedCosine9 ==
  In2 : Inport
  Discrete FIR Filter : DiscreteFir  FilterStructure=Direct form transposed  Coefficients=rcRxFilt  AccumDataTypeStr=Inherit: Same as product output
  Raised Cosine Receive Filter : commfilt2/Raised Cosine Receive Filter  Commented=on  filtType=Square root  R=0.2  filtSpan=40  N=4  downFactor=1  downOffset=0  filterGain=1  InputProcessing=Columns as channels (frame based)  RateOptions=Enforce single-rate processing  framing=Mute  checkCoeff=on  variableName=rcRxFilt  currentFiltSpan=40  D=(40)/2  inputOffset=0  sampMode=Mute  saveAsFlag=0  rateMode=Downsampling  checkGain=Normalized  launchFVT=on  roundingMode=Floor  overflowMode=off  coeffDataTypeStr=Inherit: Same word length as input  coeffMin=[]  coeffMax=[]  coeffLastDataTypeStr=Inherit: Same word length as input  accumDataTypeStr=Inherit: Same as product output  accumLastDataTypeStr=Inherit: Same as product output  outputDataTypeStr=Inherit: Same as accumulator  outputMin=[]  outputMax=[]  outputLastDataTypeStr=Inherit: Same as accumulator
  Out2 : Outport
  wires:
  Discrete FIR Filter/1 -> Out2/1
  In2/1 -> Discrete FIR Filter/1
